simulink model "r_axis_pid_ff_traj"  (R2024b)
settings: Solver=ode4  StartTime=0.0  StopTime=simulation_time  FixedStep=Ts  RelTol=1e-3
undefined symbols (not defined in the file): b_r, Kd_r, Ki_r, Kp_r, m_r, r_final, r_initial, simulation_time, Ts
libraries: slpidlib x1
settings Model: Creator=dell  LastModifiedBy=dell

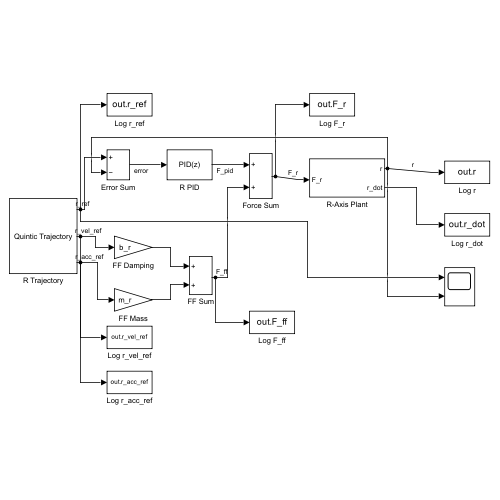
[thumbnail: Simulink's stored preview of the top-level diagram]
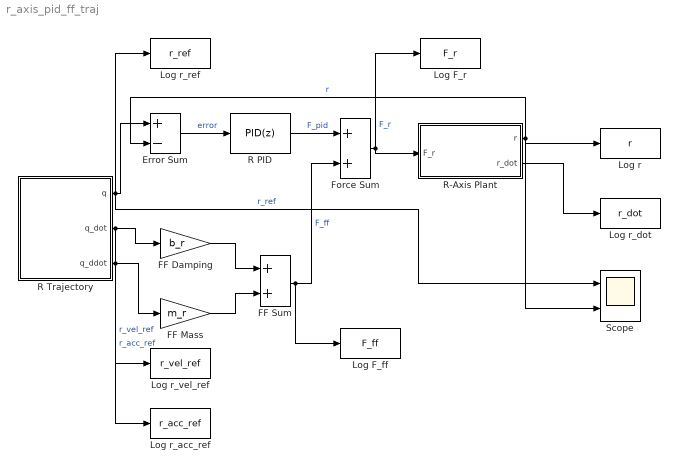
== system r_axis_pid_ff_traj ==
  Error Sum : Sum  Inputs=+-
  FF Damping : Gain  Gain=b_r
  FF Mass : Gain  Gain=m_r
  FF Sum : Sum
  Force Sum : Sum
  Log F_ff : ToWorkspace  VariableName=F_ff  SaveFormat=Timeseries  SampleTime=-1
  Log F_r : ToWorkspace  VariableName=F_r  SaveFormat=Timeseries  SampleTime=-1
  Log r : ToWorkspace  VariableName=r  SaveFormat=Timeseries  SampleTime=-1
  Log r_acc_ref : ToWorkspace  VariableName=r_acc_ref  SaveFormat=Timeseries  SampleTime=-1
  Log r_dot : ToWorkspace  VariableName=r_dot  SaveFormat=Timeseries  SampleTime=-1
  Log r_ref : ToWorkspace  VariableName=r_ref  SaveFormat=Timeseries  SampleTime=-1
  Log r_vel_ref : ToWorkspace  VariableName=r_vel_ref  SaveFormat=Timeseries  SampleTime=-1
  R PID : slpidlib/PID Controller  Controller=PID  Form=Parallel  TimeDomain=Discrete-time  UseExternalTs=off  SampleTime=Ts  IntegratorMethod=Backward Euler  FilterMethod=Forward Euler  ControllerParametersSource=internal  P=Kp_r  I=Ki_r  UseKiTs=off  D=Kd_r  UseExternalDerivativeSource=off  N=100  UseFilter=off  TunerSelectOption=Transfer Function Based (PID Tuner App)  InitialConditionSource=internal  InitialConditionForIntegrator=0  InitialConditionForFilter=0  DifferentiatorICPrevScaledInput=0  ExternalReset=none  TrackingMode=off  Kt=1  LimitOutput=off  SatLimitsSource=internal  UpperSaturationLimit=inf  LowerSaturationLimit=-inf  LinearizeAsGain=off  AntiWindupMode=none  Kb=1  LimitIntegrator=off  UpperIntegratorSaturationLimit=inf  LowerIntegratorSaturationLimit=-inf  POutMin=[]  POutMax=[]  IOutMin=[]  IOutMax=[]  DOutMin=[]  DOutMax=[]  NOutMin=[]  NOutMax=[]  SumOutMin=[]  SumOutMax=[]  SaturationOutMin=[]  SaturationOutMax=[]  PParamMin=[]  PParamMax=[]  IParamMin=[]  IParamMax=[]  DParamMin=[]  DParamMax=[]  NParamMin=[]  NParamMax=[]  KbParamMin=[]  KbParamMax=[]  KtParamMin=[]  KtParamMax=[]  KbOutMin=[]  KbOutMax=[]  KtOutMin=[]  KtOutMax=[]  IntegratorOutMin=[]  IntegratorOutMax=[]  FilterOutMin=[]  FilterOutMax=[]  SumI1OutMin=[]  SumI1OutMax=[]  SumI2OutMin=[]  SumI2OutMax=[]  SumI3OutMin=[]  SumI3OutMax=[]  SumI4OutMin=[]  SumI4OutMax=[]  SumDOutMin=[]  SumDOutMax=[]  DifferentiatorOutMin=[]  DifferentiatorOutMax=[]  FilterDiffOutCoefMin=[]  FilterDiffOutCoefMax=[]  ReciprocalOutMin=[]  ReciprocalOutMax=[]  SumDenOutMin=[]  SumDenOutMax=[]  SumNumOutMin=[]  SumNumOutMax=[]  DivideOutMin=[]  DivideOutMax=[]  UdiffTsProdOutMin=[]  UdiffTsProdOutMax=[]  NTsProdOutMin=[]  NTsProdOutMax=[]  UintegralTsProdOutMin=[]  UintegralTsProdOutMax=[]  UngainTsProdOutMin=[]  UngainTsProdOutMax=[]  ClampingZeroOutDataTypeStr=Inherit: Inherit via back propagation  ClampingZeroOutMin=[]  ClampingZeroOutMax=[]  FilterDenConstantOutDataTypeStr=Inherit: Inherit via back propagation  FilterDenConstantOutMin=[]  FilterDenConstantOutMax=[]  PCopyOutDataTypeStr=Inherit: Inherit via back propagation  PCopyOutMin=[]  PCopyOutMax=[]  NCopyOutDataTypeStr=Inherit: Inherit via back propagation  NCopyOutMin=[]  NCopyOutMax=[]  IntegratorContinuousStateAttributes=''  IntegratorStateMustResolveToSignalObject=off  IntegratorRTWStateStorageClass=Auto  FilterContinuousStateAttributes=''  FilterStateMustResolveToSignalObject=off  FilterRTWStateStorageClass=Auto  ParallelPVariant=InternalParameters  IdealPVariant=Disabled  IVariant=InternalParameters  DVariant=InternalParameters  IntegratorVariant=Discrete  SatVariant=Disabled  AWVariant=Passthrough  PCopyVariant=Disabled  TRVariant=Disabled  FdbkBlocksVariant=Forward  IdealPFdbkVariant=Disabled  SatFdbkVariant=Disabled  DerivativeFilterVariant=Differentiator  NVariant=Passthrough  NCopyVariant=Disabled_SignalSpec  FilterICVariant=InternalICsDifferentiator  IntegratorICVariant=InternalICs  ExternalResetVariant=Disabled  TRSumVariant=Passthrough  SumFdbkVariant=Disabled  SumVariant=Sum_PID  TsampFilterVariant=InternalTs  TsampNgainVariant=Passthrough  TsampIntegralVariant=Disabled_SignalSpec  ExternalSaturationOutDataTypeStr=Inherit: Same as second input  DerivativeSourceVariant=ErrorSignal  PreIntVariant=InternalPreInt
      settings: LibrarySourceBlock=simulink/Discrete/Discrete PID Controller
  R Trajectory : Subsystem  mask(Quintic Trajectory){q0=r_initial, qf=r_final, T=simulation_time}
      mask prompts: q0 "Start position q0"; qf "Final position qf"; T "Duration T (s)"
      mask help: Rest-to-rest quintic trajectory from q0 to qf over T seconds. Outputs position, velocity and acceleration.
      mask Display: disp('Quintic Trajectory')
  R-Axis Plant : Subsystem
  Scope : Scope  NumInputPorts=2
  wires:
  Error Sum/1 -> R PID/1  "error"
  R PID/1 -> Force Sum/1  "F_pid"
  FF Damping/1 -> FF Sum/1
  FF Mass/1 -> FF Sum/2
  FF Sum/1 -> Force Sum/2, Log F_ff/1  "F_ff"
  Force Sum/1 -> R-Axis Plant/1(F_r), Log F_r/1  "F_r"
  R-Axis Plant/1(r) -> Log r/1, Scope/2, Error Sum/2  "r"
  R-Axis Plant/2(r_dot) -> Log r_dot/1
  R Trajectory/1(q) -> Error Sum/1, Log r_ref/1, Scope/1  "r_ref"
  R Trajectory/2(q_dot) -> FF Damping/1, Log r_vel_ref/1  "r_vel_ref"
  R Trajectory/3(q_ddot) -> FF Mass/1, Log r_acc_ref/1  "r_acc_ref"

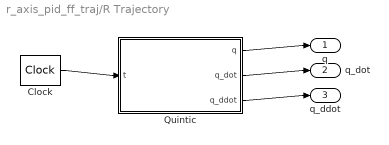
== system r_axis_pid_ff_traj/R Trajectory ==
  Clock : DigitalClock  SampleTime=Ts
  Quintic : MATLAB Function  TreatAsAtomicUnit=on
  q : Outport
  q_dot : Outport  Port=2
  q_ddot : Outport  Port=3
  wires:
  Clock/1 -> Quintic/1(t)
  Quintic/1(q) -> q/1
  Quintic/2(q_dot) -> q_dot/1
  Quintic/3(q_ddot) -> q_ddot/1

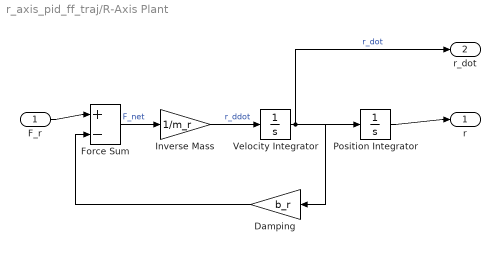
== system r_axis_pid_ff_traj/R-Axis Plant ==
  F_r : Inport
  Damping : Gain  Gain=b_r
  Force Sum : Sum  Inputs=+-
  Inverse Mass : Gain  Gain=1/m_r
  Position Integrator : Integrator  InitialCondition=r_initial
  Velocity Integrator : Integrator
  r : Outport
  r_dot : Outport  Port=2
  wires:
  F_r/1 -> Force Sum/1
  Force Sum/1 -> Inverse Mass/1  "F_net"
  Inverse Mass/1 -> Velocity Integrator/1  "r_ddot"
  Velocity Integrator/1 -> Position Integrator/1, Damping/1, r_dot/1  "r_dot"
  Damping/1 -> Force Sum/2
  Position Integrator/1 -> r/1

== matlab function r_axis_pid_ff_traj/R Trajectory/Quintic ==
  data: t input; q output; q_dot output; q_ddot output; q0 parameter; qf parameter; T parameter
function [q, q_dot, q_ddot] = quintic(t, q0, qf, T)
% Rest-to-rest quintic: zero velocity and acceleration at both ends
tau = min(max(t / T, 0), 1);
d = qf - q0;
q = q0 + d * (10*tau^3 - 15*tau^4 + 6*tau^5);
q_dot = d / T * (30*tau^2 - 60*tau^3 + 30*tau^4);
q_ddot = d / T^2 * (60*tau - 180*tau^2 + 120*tau^3);
